simulink model "Offline_DataImport_AND_ECGAnalysis_AND_SCGAnalysis"  (R2020b)
settings: Solver=FixedStepDiscrete  StartTime=0.0  StopTime=param_sim_time  FixedStep=1/fs  MaxStep=1/fs  RelTol=1e-3
undefined symbols (not defined in the file): analyses, fdesignblkfcn, fs, gcbh, param_tot_samples
libraries: dspstat3 x1
(part 4 of 5)

== system Offline_DataImport_AND_ECGAnalysis_AND_SCGAnalysis/SCG Preprocessing/Enabled SCG Preprocessing Subsystem/Filtfiltering/Bandpass Filter 1 ==
  In : Inport
  Generated Filter Block : DiscreteFir  Tag=BlockMethodSubSystem  Coefficients=[-0.0141280809748904439 0.00296128789229228515 0.00257104999710804256 0.00216178345802768047 0.00175552729414372999 0.00135185618919184472 0.000971465225508600858 0.000611761661220453987 0.000291406420521167497 4.82187739932540826e-06 -0.000231481095028417821 -0.000426883300566277893 -0.000566810793415693445 -0.000665092291782963183 -0.000708283395739488578 -0.000716103852974601593 -0.000671547633475275477 -0.000615106494933681525 -0.000488109909377643092 -0.000390234789954030728 -0.000258144491787600308 -0.000103777427082080848 3.69273719204449291e-05 0.000160217379967343004 0.000266719346682901468 0.000355855181711899407 0.00042444354991033259 0.000465107287062647284 0.000475941357662141781 0.00045436165469465474 0.000405500722307057526 0.000332653752196140906 0.000244041476717768088 0.000145867245103578971 4.31958982817989834e-05 -5.15123314384427489e-05 -0.000142923677775342456 -0.000215518203590111396 -0.000261730266501190856 -0.000295405514048500267 -0.00029258904073516806 -0.000262673662663715293 -0.000200239042161780637 -0.000119059290944066934 -1.21322536877112308e-05 0.000106963831734476281 0.00024029907401433917 0.000369441485674023434 0.000494924114257109735 0.000600074273648323539 0.000689180050721941578 0.000747556211879763649 0.000783700181000823726 0.000783037479294958205 0.000758170640681657751 0.000702221229410942768 0.00062234914182012803 0.000526336913415673471 0.000422160757970439435 0.000311595034642000654 0.000210279303290443823 0.00012116322132581063 5.51843108115603054e-05 1.14901317571792366e-05 4.63268984915096715e-07 1.97600364122418881e-05 7.52585257248264416e-05 0.000158650819102896384 0.000270390241192549133 0.000399318062573107355 0.000542643635713839848 0.000686965575031403888 0.00082909540621049771 0.000950782043587884013 0.00105531510633344837 0.0011243012388455851 0.00116225627563770577 0.00116100403898223951 0.00112659092458904618 0.00105319818945410169 0.000953344560012697739 0.000827179974613592023 0.000689621114973500843 0.000542798204792315636 0.000403935329663590928 0.000276677120819612474 0.000176948147897270508 0.000104790831399949325 7.17507496431589453e-05 7.47958920749892953e-05 0.0001189809160239471 0.000199000478147139462 0.000312036321493172272 0.000446906185270561432 0.000599958367208563298 0.000753866459386062782 0.00090376858726108622 0.00103429112272443793 0.00114049954630186627 0.00120812081357756125 0.00123691779750273109 0.00121863837734643987 0.00115823236504885609 0.00105257319614873897 0.000912433904619841529 0.000740597166721868039 0.000552884553978793408 0.000354055164106317766 0.000163199294344686802 -1.50951637483565798e-05 -0.000162513118388487796 -0.000275080946577539037 -0.000341943188723405761 -0.000363442033376501494 -0.00033415202471282282 -0.000262311282575341045 -0.000148736623332661536 -6.29165138528280099e-06 0.000158313981566005763 0.000327534481367972377 0.000492510275335960451 0.000636058676656042071 0.000750308535347654973 0.000820834153970448691 0.000843500867080383687 0.000811058974000754968 0.000725579145441419826 0.000586861203976211943 0.000405054868711680893 0.000184940546124518629 -5.5900228056928597e-05 -0.000308204861095128652 -0.000553436858002336746 -0.000780717962187617992 -0.000972296884021763008 -0.00112115970011063791 -0.00121428591472381824 -0.00125044236292902976 -0.00122449203339279784 -0.00114390543564522537 -0.00101139494448912459 -0.000841431774385854175 -0.000642541957157717614 -0.000434750691331369996 -0.000229897013949648468 -4.78783601658636093e-05 9.9539490455416782e-05 0.000197094197447343286 0.000237758271413028577 0.00021254671910410014 0.000123930849749381497 -2.84437637916960806e-05 -0.000234134053639612275 -0.000484592671067754152 -0.000762051837015052455 -0.00105285099253676732 -0.00133585896082411525 -0.00159595443115483245 -0.00181366900494322504 -0.00197783075368637359 -0.00207501327682029293 -0.00210124750065167169 -0.00205143676620881017 -0.00193252830137258941 -0.0017485276980914212 -0.00151582984003622266 ...(+13710 chars)]  InputProcessing=Columns as channels (frame based)
  Out : Outport  VectorParamsAs1DForOutWhenUnconnected=off
  wires:
  Generated Filter Block/1 -> Out/1
  In/1 -> Generated Filter Block/1

== system Offline_DataImport_AND_ECGAnalysis_AND_SCGAnalysis/SCG Preprocessing/Enabled SCG Preprocessing Subsystem/Filtfiltering/Bandpass Filter 2 ==
  In : Inport
  Generated Filter Block : DiscreteFir  Tag=BlockMethodSubSystem  Coefficients=[-0.0141280809748904439 0.00296128789229228515 0.00257104999710804256 0.00216178345802768047 0.00175552729414372999 0.00135185618919184472 0.000971465225508600858 0.000611761661220453987 0.000291406420521167497 4.82187739932540826e-06 -0.000231481095028417821 -0.000426883300566277893 -0.000566810793415693445 -0.000665092291782963183 -0.000708283395739488578 -0.000716103852974601593 -0.000671547633475275477 -0.000615106494933681525 -0.000488109909377643092 -0.000390234789954030728 -0.000258144491787600308 -0.000103777427082080848 3.69273719204449291e-05 0.000160217379967343004 0.000266719346682901468 0.000355855181711899407 0.00042444354991033259 0.000465107287062647284 0.000475941357662141781 0.00045436165469465474 0.000405500722307057526 0.000332653752196140906 0.000244041476717768088 0.000145867245103578971 4.31958982817989834e-05 -5.15123314384427489e-05 -0.000142923677775342456 -0.000215518203590111396 -0.000261730266501190856 -0.000295405514048500267 -0.00029258904073516806 -0.000262673662663715293 -0.000200239042161780637 -0.000119059290944066934 -1.21322536877112308e-05 0.000106963831734476281 0.00024029907401433917 0.000369441485674023434 0.000494924114257109735 0.000600074273648323539 0.000689180050721941578 0.000747556211879763649 0.000783700181000823726 0.000783037479294958205 0.000758170640681657751 0.000702221229410942768 0.00062234914182012803 0.000526336913415673471 0.000422160757970439435 0.000311595034642000654 0.000210279303290443823 0.00012116322132581063 5.51843108115603054e-05 1.14901317571792366e-05 4.63268984915096715e-07 1.97600364122418881e-05 7.52585257248264416e-05 0.000158650819102896384 0.000270390241192549133 0.000399318062573107355 0.000542643635713839848 0.000686965575031403888 0.00082909540621049771 0.000950782043587884013 0.00105531510633344837 0.0011243012388455851 0.00116225627563770577 0.00116100403898223951 0.00112659092458904618 0.00105319818945410169 0.000953344560012697739 0.000827179974613592023 0.000689621114973500843 0.000542798204792315636 0.000403935329663590928 0.000276677120819612474 0.000176948147897270508 0.000104790831399949325 7.17507496431589453e-05 7.47958920749892953e-05 0.0001189809160239471 0.000199000478147139462 0.000312036321493172272 0.000446906185270561432 0.000599958367208563298 0.000753866459386062782 0.00090376858726108622 0.00103429112272443793 0.00114049954630186627 0.00120812081357756125 0.00123691779750273109 0.00121863837734643987 0.00115823236504885609 0.00105257319614873897 0.000912433904619841529 0.000740597166721868039 0.000552884553978793408 0.000354055164106317766 0.000163199294344686802 -1.50951637483565798e-05 -0.000162513118388487796 -0.000275080946577539037 -0.000341943188723405761 -0.000363442033376501494 -0.00033415202471282282 -0.000262311282575341045 -0.000148736623332661536 -6.29165138528280099e-06 0.000158313981566005763 0.000327534481367972377 0.000492510275335960451 0.000636058676656042071 0.000750308535347654973 0.000820834153970448691 0.000843500867080383687 0.000811058974000754968 0.000725579145441419826 0.000586861203976211943 0.000405054868711680893 0.000184940546124518629 -5.5900228056928597e-05 -0.000308204861095128652 -0.000553436858002336746 -0.000780717962187617992 -0.000972296884021763008 -0.00112115970011063791 -0.00121428591472381824 -0.00125044236292902976 -0.00122449203339279784 -0.00114390543564522537 -0.00101139494448912459 -0.000841431774385854175 -0.000642541957157717614 -0.000434750691331369996 -0.000229897013949648468 -4.78783601658636093e-05 9.9539490455416782e-05 0.000197094197447343286 0.000237758271413028577 0.00021254671910410014 0.000123930849749381497 -2.84437637916960806e-05 -0.000234134053639612275 -0.000484592671067754152 -0.000762051837015052455 -0.00105285099253676732 -0.00133585896082411525 -0.00159595443115483245 -0.00181366900494322504 -0.00197783075368637359 -0.00207501327682029293 -0.00210124750065167169 -0.00205143676620881017 -0.00193252830137258941 -0.0017485276980914212 -0.00151582984003622266 ...(+13710 chars)]  InputProcessing=Columns as channels (frame based)
  Out : Outport  VectorParamsAs1DForOutWhenUnconnected=off
  wires:
  In/1 -> Generated Filter Block/1
  Generated Filter Block/1 -> Out/1

== system Offline_DataImport_AND_ECGAnalysis_AND_SCGAnalysis/SCG Preprocessing/Enabled SCG Preprocessing Subsystem/To Workspace: Processed SCGxyz/To Workspace SCG Enabled Subsystem ==
  note: The subsystem is only enabled when it receives a (non-zero) signal
  In1 : Inport
  Enable : EnablePort
  To Workspace SCG : ToWorkspace  VariableName=out_scg_xyz_preprocessing  SaveFormat=Structure  SampleTime=-1
  wires:
  In1/1 -> To Workspace SCG/1

== system Offline_DataImport_AND_ECGAnalysis_AND_SCGAnalysis/SCG Analysis/Enabled SCG Analysis Subsystem/Anisotropy Characterization/Average Cycle Max Diameter//Volume Calculator/SCG xyz Average Cycle ==
  in_ecg_r : Inport
  in_scg_xyz : Inport  Port=2
  Average SCGxyz Cycle Calculator : MATLAB Function  TreatAsAtomicUnit=on
  Constant : Constant
  Fixed-Size Converter 2 : Selector  NumberOfDimensions=2  IndexOptions=Starting and ending indices (port),Index vector (dialog)  Indices=[1:min(analyses.ecg.RR)],[1 2 3]  OutputSizes=1,1
  Min RR Calculator : MATLAB Function  TreatAsAtomicUnit=on
  Mux : Mux  Inputs=2
  out_scg_xyz_avgcycle : Outport  VectorParamsAs1DForOutWhenUnconnected=off
  wires:
  in_scg_xyz/1 -> Average SCGxyz Cycle Calculator/2(scgxyz)
  in_ecg_r/1 -> Min RR Calculator/1(r_pos), Average SCGxyz Cycle Calculator/1(r_pos)
  Average SCGxyz Cycle Calculator/1(scgxyz_avgcycle) -> Fixed-Size Converter 2/1
  Fixed-Size Converter 2/1 -> out_scg_xyz_avgcycle/1
  Constant/1 -> Mux/1
  Min RR Calculator/1(min_rr) -> Mux/2
  Mux/1 -> Fixed-Size Converter 2/2

== system Offline_DataImport_AND_ECGAnalysis_AND_SCGAnalysis/SCG Analysis/Enabled SCG Analysis Subsystem/Anisotropy Characterization/Average Cycle Max//Median Diameter Calculator/SCG xyz Average Cycle ==
  in_ecg_r : Inport
  in_scg_xyz : Inport  Port=2
  Average SCGxyz Cycle Calculator : MATLAB Function  TreatAsAtomicUnit=on
  Constant : Constant
  Fixed-Size Converter 2 : Selector  NumberOfDimensions=2  IndexOptions=Starting and ending indices (port),Index vector (dialog)  Indices=[1:min(analyses.ecg.RR)],[1 2 3]  OutputSizes=1,1
  Min RR Calculator : MATLAB Function  TreatAsAtomicUnit=on
  Mux : Mux  Inputs=2
  out_scg_xyz_avgcycle : Outport  VectorParamsAs1DForOutWhenUnconnected=off
  wires:
  in_scg_xyz/1 -> Average SCGxyz Cycle Calculator/2(scgxyz)
  in_ecg_r/1 -> Min RR Calculator/1(r_pos), Average SCGxyz Cycle Calculator/1(r_pos)
  Average SCGxyz Cycle Calculator/1(scgxyz_avgcycle) -> Fixed-Size Converter 2/1
  Fixed-Size Converter 2/1 -> out_scg_xyz_avgcycle/1
  Constant/1 -> Mux/1
  Min RR Calculator/1(min_rr) -> Mux/2
  Mux/1 -> Fixed-Size Converter 2/2

== system Offline_DataImport_AND_ECGAnalysis_AND_SCGAnalysis/SCG Analysis/Enabled SCG Analysis Subsystem/Anisotropy Characterization/Average Cycle Max//Min Diameter Calculator/SCG xyz Average Cycle ==
  in_ecg_r : Inport
  in_scg_xyz : Inport  Port=2
  Average SCGxyz Cycle Calculator : MATLAB Function  TreatAsAtomicUnit=on
  Constant : Constant
  Fixed-Size Converter 2 : Selector  NumberOfDimensions=2  IndexOptions=Starting and ending indices (port),Index vector (dialog)  Indices=[1:min(analyses.ecg.RR)],[1 2 3]  OutputSizes=1,1
  Min RR Calculator : MATLAB Function  TreatAsAtomicUnit=on
  Mux : Mux  Inputs=2
  out_scg_xyz_avgcycle : Outport  VectorParamsAs1DForOutWhenUnconnected=off
  wires:
  Mux/1 -> Fixed-Size Converter 2/2
  Min RR Calculator/1(min_rr) -> Mux/2
  Constant/1 -> Mux/1
  Fixed-Size Converter 2/1 -> out_scg_xyz_avgcycle/1
  Average SCGxyz Cycle Calculator/1(scgxyz_avgcycle) -> Fixed-Size Converter 2/1
  in_ecg_r/1 -> Average SCGxyz Cycle Calculator/1(r_pos), Min RR Calculator/1(r_pos)
  in_scg_xyz/1 -> Average SCGxyz Cycle Calculator/2(scgxyz)

== system Offline_DataImport_AND_ECGAnalysis_AND_SCGAnalysis/SCG Analysis/Enabled SCG Analysis Subsystem/Signal Generation/2DMod Calculator/2DMod Calculator ==
  2D Components : Inport
  Square Root1 : Sqrt  SaturateOnIntegerOverflow=on
  Square1 : Math  Operator=square  SignedPower=on  SaturateOnIntegerOverflow=on
  Sum1 : Sum  Inputs=+  CollapseMode=Specified dimension  CollapseDim=2
  2D Modulus : Outport  VectorParamsAs1DForOutWhenUnconnected=off
  wires:
  Square1/1 -> Sum1/1
  Sum1/1 -> Square Root1/1
  2D Components/1 -> Square1/1
  Square Root1/1 -> 2D Modulus/1

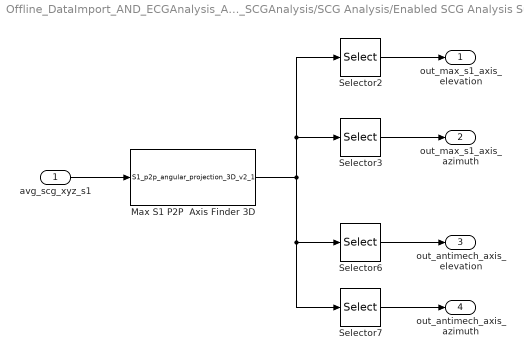
== system Offline_DataImport_AND_ECGAnalysis_AND_SCGAnalysis/SCG Analysis/Enabled SCG Analysis Subsystem/Signal Generation/3D Projections/3D Max S1 p2p Axis Calculator ==
  avg_scg_xyz_s1 : Inport
  Max S1 P2P  Axis Finder 3D : MATLABFcn  MATLABFcn=S1_p2p_angular_projection_3D_v2_1  OutputDimensions=4  Output1D=off
  Selector2 : Selector  InputPortWidth=4  IndexOptions=Index vector (dialog)  Indices=[1]  OutputSizes=1
  Selector3 : Selector  InputPortWidth=4  IndexOptions=Index vector (dialog)  Indices=[2]  OutputSizes=1
  Selector6 : Selector  InputPortWidth=4  IndexOptions=Index vector (dialog)  Indices=[3]  OutputSizes=1
  Selector7 : Selector  InputPortWidth=4  IndexOptions=Index vector (dialog)  Indices=[4]  OutputSizes=1
  out_max_s1_axis_elevation : Outport
  out_max_s1_axis_azimuth : Outport  Port=2
  out_antimech_axis_elevation : Outport  Port=3
  out_antimech_axis_azimuth : Outport  Port=4
  wires:
  avg_scg_xyz_s1/1 -> Max S1 P2P  Axis Finder 3D/1
  Max S1 P2P  Axis Finder 3D/1 -> Selector7/1, Selector6/1, Selector2/1, Selector3/1
  Selector2/1 -> out_max_s1_axis_elevation/1
  Selector3/1 -> out_max_s1_axis_azimuth/1
  Selector7/1 -> out_antimech_axis_azimuth/1
  Selector6/1 -> out_antimech_axis_elevation/1

== system Offline_DataImport_AND_ECGAnalysis_AND_SCGAnalysis/SCG Analysis/Enabled SCG Analysis Subsystem/Signal Generation/3D Projections/3D Mechanical Axis Calculator ==
  in_avg_scg_xyz_s1 : Inport
  Cardiac Mechanical Systolic Axis Finder 3D : MATLABFcn  MATLABFcn=cardiac_mech_systolic_axis_finder_3D  OutputDimensions=4  Output1D=off
  Selector : Selector  InputPortWidth=4  IndexOptions=Index vector (dialog)  Indices=[1]  OutputSizes=1
  Selector1 : Selector  InputPortWidth=4  IndexOptions=Index vector (dialog)  Indices=[2]  OutputSizes=1
  Selector4 : Selector  InputPortWidth=4  IndexOptions=Index vector (dialog)  Indices=[3]  OutputSizes=1
  Selector5 : Selector  InputPortWidth=4  IndexOptions=Index vector (dialog)  Indices=[4]  OutputSizes=1
  out_mech_axis_elevation : Outport
  out_mech_axis_azimuth : Outport  Port=2
  out_antimech_axis_elevation : Outport  Port=3
  out_antimech_axis_azimuth : Outport  Port=4
  wires:
  Cardiac Mechanical Systolic Axis Finder 3D/1 -> Selector5/1, Selector4/1, Selector/1, Selector1/1
  Selector5/1 -> out_antimech_axis_azimuth/1
  Selector/1 -> out_mech_axis_elevation/1
  Selector4/1 -> out_antimech_axis_elevation/1
  Selector1/1 -> out_mech_axis_azimuth/1
  in_avg_scg_xyz_s1/1 -> Cardiac Mechanical Systolic Axis Finder 3D/1

== system Offline_DataImport_AND_ECGAnalysis_AND_SCGAnalysis/SCG Analysis/Enabled SCG Analysis Subsystem/Signal Generation/3D Projections/SCG xyz Average Cycle ==
  in_ecg_r : Inport
  in_scg_xyz : Inport  Port=2
  Average SCGxyz Cycle Calculator : MATLAB Function  TreatAsAtomicUnit=on
  Constant : Constant
  Fixed-Size Converter 2 : Selector  NumberOfDimensions=2  IndexOptions=Starting and ending indices (port),Index vector (dialog)  Indices=[1:min(analyses.ecg.RR)],[1 2 3]  OutputSizes=1,1
  Min RR Calculator : MATLAB Function  TreatAsAtomicUnit=on
  Mux : Mux  Inputs=2
  out_scg_xyz_avgcycle : Outport  VectorParamsAs1DForOutWhenUnconnected=off
  wires:
  in_scg_xyz/1 -> Average SCGxyz Cycle Calculator/2(scgxyz)
  in_ecg_r/1 -> Min RR Calculator/1(r_pos), Average SCGxyz Cycle Calculator/1(r_pos)
  Average SCGxyz Cycle Calculator/1(scgxyz_avgcycle) -> Fixed-Size Converter 2/1
  Fixed-Size Converter 2/1 -> out_scg_xyz_avgcycle/1
  Constant/1 -> Mux/1
  Min RR Calculator/1(min_rr) -> Mux/2
  Mux/1 -> Fixed-Size Converter 2/2

== matlab function Offline_DataImport_AND_ECGAnalysis_AND_SCGAnalysis/SCG Analysis/Enabled SCG Analysis Subsystem/Signal Generation/3D Projections/MATLAB Function1 ==
  data: scg_xyz input; el_scg input size=[1]; projection output size=[param_tot_samples 1]; az_scg input size=[1]
function projection = slk_axis_projection(scg_xyz, el_scg, az_scg)

el_mat = el_scg;
az_mat = -1*az_scg;

[xhat_mat, yhat_mat, zhat_mat] = sph2cart(az_mat*pi/180,el_mat*pi/180,1);
% Converting to the SCG convention reference frame (this depends on the accelerometer and its placement orientation! - they should be such that they match the conventional SCG reference frame).
xhat_scg = xhat_mat;
yhat_scg = zhat_mat;
zhat_scg = -1*yhat_mat;

projection_axis = [xhat_scg yhat_scg zhat_scg];
    
projection = zeros(size(scg_xyz,1),1);
    
for i=1:size(scg_xyz,1)
    
    projection(i) = dot(scg_xyz(i,:),projection_axis);
    
end

figure;
ax = [0 0 0 0];

ax(1) = subplot(4,1,1); plot(scg_xyz(:,1),'b'); title('x'); box off; ylabel('Acceleration (mg)');
ax(2) = subplot(4,1,2); plot(scg_xyz(:,2),'b'); title('y'); box off; ylabel('Acceleration (mg)');
ax(3) = subplot(4,1,3); plot(scg_xyz(:,3),'b'); title('z'); box off; ylabel('Acceleration (mg)');
ax(4) = subplot(4,1,4); plot(projection,'r'); title('Antimechanical Axis Projection'); box off; ylabel('Acceleration (mg)');
xlabel('Sample no.')
linkaxes(ax,'xy')
end

== matlab function Offline_DataImport_AND_ECGAnalysis_AND_SCGAnalysis/SCG Analysis/Enabled SCG Analysis Subsystem/Signal Generation/3D Projections/MATLAB Function2 ==
  data: scg_xyz input; el_scg input size=[1]; projection output size=[param_tot_samples 1]; az_scg input size=[1]
function projection = slk_axis_projection(scg_xyz, el_scg, az_scg)

el_mat = el_scg;
az_mat = -1*az_scg;

[xhat_mat, yhat_mat, zhat_mat] = sph2cart(az_mat*pi/180,el_mat*pi/180,1);
% Converting to the SCG convention reference frame (this depends on the accelerometer and its placement orientation! - they should be such that they match the conventional SCG reference frame).
xhat_scg = xhat_mat;
yhat_scg = zhat_mat;
zhat_scg = -1*yhat_mat;

projection_axis = [xhat_scg yhat_scg zhat_scg];
    
projection = zeros(size(scg_xyz,1),1);
    
for i=1:size(scg_xyz,1)
    
    projection(i) = dot(scg_xyz(i,:),projection_axis);
    
end

figure;
ax = [0 0 0 0];

ax(1) = subplot(4,1,1); plot(scg_xyz(:,1),'b'); title('x'); box off; ylabel('Acceleration (mg)');
ax(2) = subplot(4,1,2); plot(scg_xyz(:,2),'b'); title('y'); box off; ylabel('Acceleration (mg)');
ax(3) = subplot(4,1,3); plot(scg_xyz(:,3),'b'); title('z'); box off; ylabel('Acceleration (mg)');
ax(4) = subplot(4,1,4); plot(projection,'g'); title('Max S1 P2P Axis Projection'); box off; ylabel('Acceleration (mg)');
xlabel('Sample no.')
linkaxes(ax,'xy')
end

== matlab function Offline_DataImport_AND_ECGAnalysis_AND_SCGAnalysis/SCG Analysis/Enabled SCG Analysis Subsystem/Signal Generation/3D Projections/MATLAB Function3 ==
  data: scg_xyz input; el_scg input size=[1]; projection output size=[param_tot_samples 1]; az_scg input size=[1]
function projection = slk_axis_projection(scg_xyz, el_scg, az_scg)

el_mat = el_scg;
az_mat = -1*az_scg;

[xhat_mat, yhat_mat, zhat_mat] = sph2cart(az_mat*pi/180,el_mat*pi/180,1);
% Converting to the SCG convention reference frame (this depends on the accelerometer and its placement orientation! - they should be such that they match the conventional SCG reference frame).
xhat_scg = xhat_mat;
yhat_scg = zhat_mat;
zhat_scg = -1*yhat_mat;

projection_axis = [xhat_scg yhat_scg zhat_scg];
    
projection = zeros(size(scg_xyz,1),1);
    
for i=1:size(scg_xyz,1)
    
    projection(i) = dot(scg_xyz(i,:),projection_axis);
    
end

figure;
ax = [0 0 0 0];

ax(1) = subplot(4,1,1); plot(scg_xyz(:,1),'b'); title('x'); box off; ylabel('Acceleration (mg)');
ax(2) = subplot(4,1,2); plot(scg_xyz(:,2),'b'); title('y'); box off; ylabel('Acceleration (mg)');
ax(3) = subplot(4,1,3); plot(scg_xyz(:,3),'b'); title('z'); box off; ylabel('Acceleration (mg)');
ax(4) = subplot(4,1,4); plot(projection,'r'); title('Min S1 P2P Axis Projection'); box off; ylabel('Acceleration (mg)');
xlabel('Sample no.')
linkaxes(ax,'xy')
end

== matlab function Offline_DataImport_AND_ECGAnalysis_AND_SCGAnalysis/ECG Analysis/Enabled ECG Analysis Subsystem/Assign To Workspace: Num Cycles/Enabled To Workspace ECG Num Cycles/Slk Wrapped Assigned To Workspace ==
  data: assigned_var input size=[1]
function slk_wrapped_assign_to_workspace(assigned_var)
% Wrapped simulink function to assign an input 'assigned_var' to the base workspace.

coder.extrinsic('assign_num_cycles_to_workspace');

if assigned_var % Only go into the function if a valid variable is passed to it.
    assign_num_cycles_to_workspace(assigned_var)
end

end

== matlab function Offline_DataImport_AND_ECGAnalysis_AND_SCGAnalysis/ECG Analysis/Enabled ECG Analysis Subsystem/Assign To Workspace: ECG PQRST/Enabled To Workspace ECG PQRST/Slk Wrapped Assigned to Workspace ==
  data: ecg_pqrst input size=[4*ceil(param_sim_time) 5]
function slk_wrapped_assign_to_workspace(ecg_pqrst)
% Wrapped simulink function to assign an input 'assigned_var' to the base workspace.

coder.extrinsic('assign_ecg_pqrst_to_workspace');

if ecg_pqrst(:,3) % Only go into the function if a valid ECG R pos sequence is passed to it.
    assign_ecg_pqrst_to_workspace(ecg_pqrst);
end

end
